simulink model "busdemo"  (Simulink 6.0)
settings: Solver=VariableStepDiscrete  StartTime=0.0  StopTime=10  MaxStep=.05  RelTol=1e-3
libraries: simulink x1
settings Model: CovMetricSettings=d  Creator=The MathWorks Inc.  LastModifiedBy=batserve  ExtModeTrigMode=oneshot  ExtModeArmWhenConnect=off  ExtModeAutoUpdateStatusClock=off
settings DataIOCC: LimitDataPoints=off
settings OptimizationCC: BlockReduction=off  BooleanDataType=off
settings DebuggingCC: CheckExecutionContextPreStartOutputMsg=on  CheckExecutionContextRuntimeOutputMsg=on  SolverPrmCheckMsg=none  IntegerOverflowMsg=none
settings HardwareCC: TargetUnknown=on

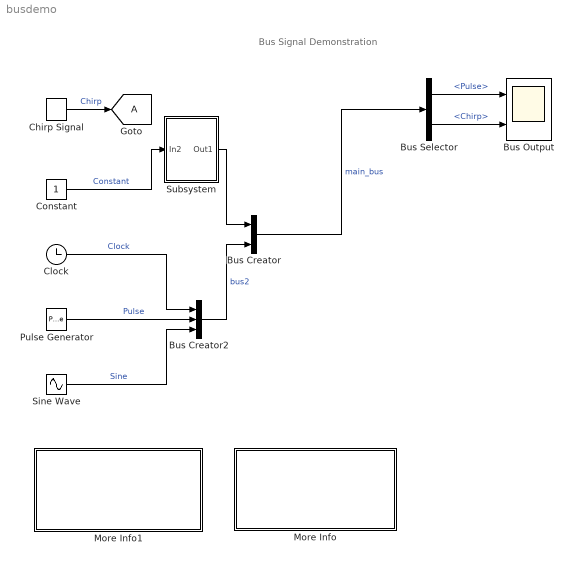
== system busdemo ==
  note: Bus Signal Demonstration
  Bus Creator : BusCreator  DialogController=Simulink.DDGSource_Bus  Inputs=2
  Bus Creator2 : BusCreator  DialogController=Simulink.DDGSource_Bus  Inputs=3
  Bus Selector : BusSelector  DialogController=Simulink.DDGSource_Bus  OutputSignals=bus2.Pulse,bus1.Chirp
  Bus Output : Scope  NumInputPorts=2
      settings: StartFcn=open_system(gcbh)  TimeRange=10  YMin=-3~-5  YMax=3~5  DataFormat=Structure
  Chirp Signal : simulink/Sources/Chirp Signal  f1=0.1  T=10  f2=5
  Clock : Clock
      settings: Decimation=10
  Constant : Constant
  More Info : Subsystem  PropExecContextAcrossSSBoundary=on
      settings: OpenFcn=busdemoscript
      mask Display: disp('Double click here \nfor a step-by-step\ntutorial on this model.')
  More Info1 : Subsystem  PropExecContextAcrossSSBoundary=on
      settings: OpenFcn=simcad(bdroot);
      mask Display: disp('Double click\nhere for general\nSimulink Help')
  Pulse Generator : DiscretePulseGenerator
  Sine Wave : Sin  SampleTime=0
  Subsystem : Subsystem  PropExecContextAcrossSSBoundary=on
  tag scope: A=global
  wires:
  Clock/1 -> Bus Creator2/1  "Clock"
  Pulse Generator/1 -> Bus Creator2/2  "Pulse"
  Sine Wave/1 -> Bus Creator2/3  "Sine"
  Constant/1 -> Subsystem/1(In2)  "Constant"
  Bus Creator/1 -> Bus Selector/1  "main_bus"
  Bus Selector/1 -> Bus Output/1  "<Pulse>"
  Bus Selector/2 -> Bus Output/2  "<Chirp>"
  Subsystem/1(Out1) -> Bus Creator/1
  Bus Creator2/1 -> Bus Creator/2  "bus2"
  Chirp Signal/1 -> [A]  "Chirp"

== system busdemo/More Info ==
  note: This demonstration shows how signals may be grouped and ungrouped while
      | retaining their names.  In this demonstration, 5 signals are created and labelled
      | appropriately.  These signals are then mux'd together to create a bus of signals.
      | This bus of signals is then fed into the Bus Selector block.  Inside of the Bus
      | Selector block, the Pulse and Chirp signals are chosen to be output from the
      | original signal bus.
      |
      | It is possible to place a nest signal buses and then still retrieve the original signal
      | with its label.
  note: Bus Block Demonstration

== system busdemo/More Info1 ==

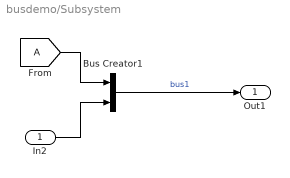
== system busdemo/Subsystem ==
  In2 : Inport  Port=1  LatchInput=off
  Bus Creator1 : BusCreator  DialogController=Simulink.DDGSource_Bus  Inputs=2
  Out1 : Outport
  wires:
  [A] -> Bus Creator1/1
  Bus Creator1/1 -> Out1/1  "bus1"
  In2/1 -> Bus Creator1/2
